simulink model "extended_state_observor_pendulum"  (R2019b)
settings: Solver=FixedStepAuto  StartTime=0.0  StopTime=20  FixedStep=0.001  RelTol=1e-3
values from neighbouring files (symbols this model uses):
  K = acker(A,B,poles_control)    [eso_design.m]
  L = [3*wd 3*wd^2 wd^3]'    [eso_design.m]
  wn = 1    [eso_design.m]
  zeta = 0.1    [eso_design.m]
settings Model: Creator=henry  LastModifiedBy=henry

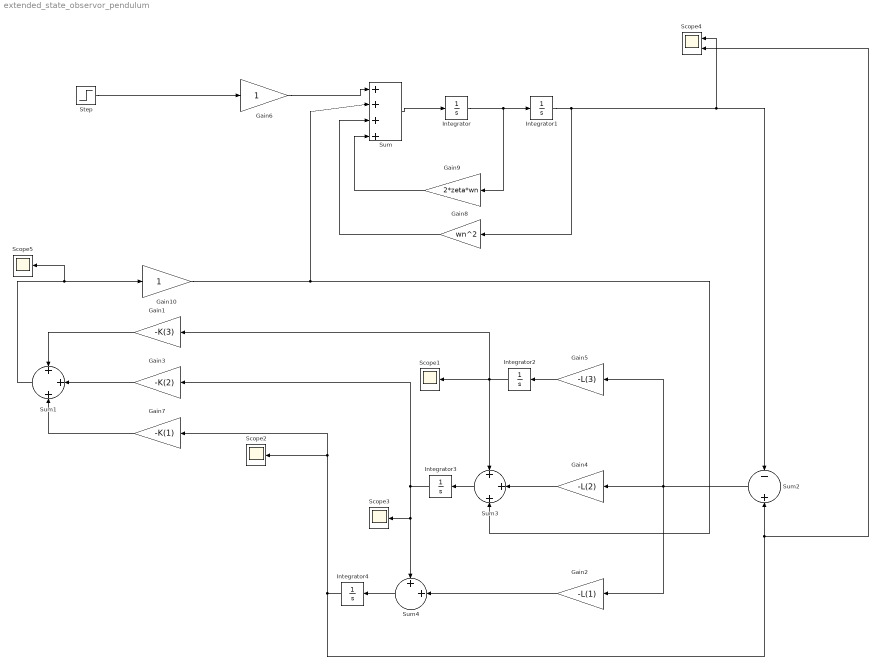
== system extended_state_observor_pendulum ==
  Gain1 : Gain  Gain=-K(3)
  Gain10 : Gain
  Gain2 : Gain  Gain=-L(1)
  Gain3 : Gain  Gain=-K(2)
  Gain4 : Gain  Gain=-L(2)
  Gain5 : Gain  Gain=-L(3)
  Gain6 : Gain
  Gain7 : Gain  Gain=-K(1)
  Gain8 : Gain  Gain=wn^2
  Gain9 : Gain  Gain=2*zeta*wn
  Integrator : Integrator  InitialCondition=-1.5
  Integrator1 : Integrator  InitialCondition=0.5
  Integrator2 : Integrator
  Integrator3 : Integrator
  Integrator4 : Integrator
  Scope{1..3,5} (4 alike) : Scope
  Scope4 : Scope  NumInputPorts=2
  Step : Step  Time=5  SampleTime=0
  Sum : Sum  Inputs=|++++
  Sum1 : Sum  Inputs=+|+|+
  Sum2 : Sum  Inputs=-|+
  Sum3 : Sum  Inputs=+|+|+
  Sum4 : Sum  Inputs=++|
  wires:
  Sum/1 -> Integrator/1
  Integrator/1 -> Gain9/1, Integrator1/1
  Sum2/1 -> Gain5/1, Gain2/1, Gain4/1
  Gain2/1 -> Sum4/2
  Gain4/1 -> Sum3/2
  Gain5/1 -> Integrator2/1
  Integrator2/1 -> Gain1/1, Scope1/1, Sum3/1
  Sum3/1 -> Integrator3/1
  Integrator3/1 -> Gain3/1, Scope3/1, Sum4/1
  Sum4/1 -> Integrator4/1
  Integrator4/1 -> Gain7/1, Scope2/1, Scope4/2, Sum2/2
  Sum1/1 -> Scope5/1, Gain10/1
  Integrator1/1 -> Gain8/1, Scope4/1, Sum2/1
  Gain6/1 -> Sum/1
  Step/1 -> Gain6/1
  Gain8/1 -> Sum/3
  Gain7/1 -> Sum1/3
  Gain3/1 -> Sum1/2
  Gain1/1 -> Sum1/1
  Gain9/1 -> Sum/4
  Gain10/1 -> Sum/2, Sum3/3
